simulink model "controlledplant"  (R2016b)
settings: Solver=VariableStepAuto  StartTime=0.0  StopTime=stoptime  RelTol=1e-3
values from neighbouring files (symbols this model uses):
  A = [0.2 0.7 ... (first row only)    [main.m]
  B = [0.1 0.5]'    [main.m]
  d = p*0.1    (= 0.1)    [runMPC.m]
  Delta = p*0.05    (= 0.05)    [runMPC.m]
  Delta0 = [do.Data(end,:)]'    [runMPC.m]
  m = 1    [main.m]
  n = 2    [main.m]
  stepsize = 1e-4    (= 0.0001)    [main.m]
  x0 = x.Data(end,:)'-Delta0    [runMPC.m]
libraries: simulink x2
settings Model: Creator=Berk  LastModifiedBy=Berk

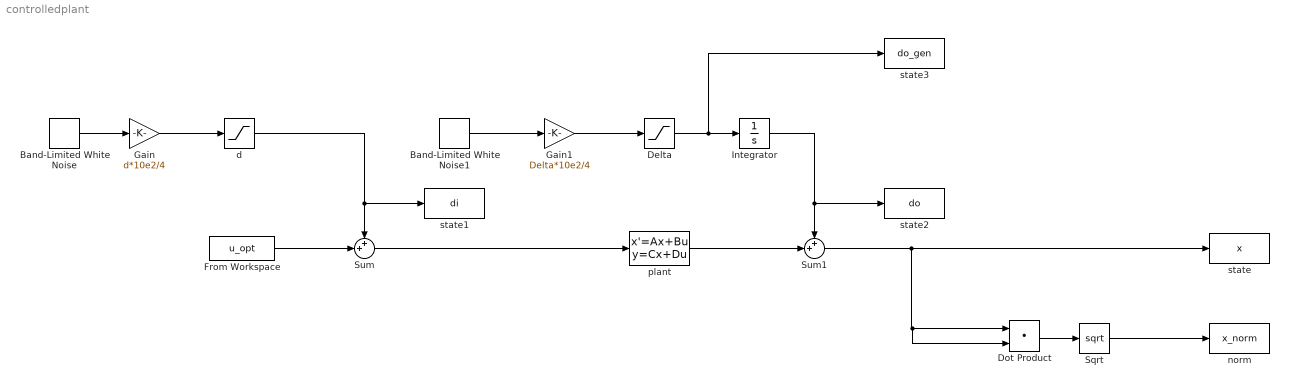
== system controlledplant ==
  Band-Limited White Noise : simulink/Sources/Band-Limited White Noise  Cov=1e-10  Ts=stepsize  seed=randi(20000)
  Band-Limited White Noise1 : simulink/Sources/Band-Limited White Noise  Cov=1e-10  Ts=stepsize  seed=randi(7500)
  Delta : Saturate  UpperLimit=Delta  LowerLimit=-Delta
  Dot Product : DotProduct  InputSameDT=on  OutDataTypeStr=Inherit: Inherit via internal rule
  From Workspace : FromWorkspace  VariableName=u_opt  SampleTime=0
  Gain : Gain  Gain=d*10e2/4
  Gain1 : Gain  Gain=Delta*10e2/4
  Integrator : Integrator  InitialCondition=Delta0
  Sqrt : Sqrt  SaturateOnIntegerOverflow=on
  Sum : Sum  Inputs=++|
  Sum1 : Sum  Inputs=++|
  d : Saturate  UpperLimit=d  LowerLimit=-d
  norm : ToWorkspace  VariableName=x_norm  SaveFormat=Timeseries  SampleTime=-1
  plant : StateSpace  A=A  B=B  C=eye(n)  D=zeros(n,m)  X0=x0
  state : ToWorkspace  VariableName=x  SaveFormat=Timeseries  SampleTime=-1
  state1 : ToWorkspace  VariableName=di  SaveFormat=Timeseries  SampleTime=-1
  state2 : ToWorkspace  VariableName=do  SaveFormat=Timeseries  SampleTime=-1
  state3 : ToWorkspace  VariableName=do_gen  SaveFormat=Timeseries  SampleTime=-1
  wires:
  From Workspace/1 -> Sum/2
  Sum/1 -> plant/1
  Integrator/1 -> state2/1, Sum1/1
  plant/1 -> Sum1/2
  Sqrt/1 -> norm/1
  Sum1/1 -> Dot Product/2, Dot Product/1, state/1
  Dot Product/1 -> Sqrt/1
  d/1 -> state1/1, Sum/1
  Band-Limited White Noise/1 -> Gain/1
  Gain/1 -> d/1
  Delta/1 -> state3/1, Integrator/1
  Band-Limited White Noise1/1 -> Gain1/1
  Gain1/1 -> Delta/1
